simulink model "Scara"  (R2016b)
settings: Solver=VariableStepAuto  StartTime=0.0  StopTime=15.0  RelTol=1e-3
settings Model: Creator=Roozbeh  LastModifiedBy=Roozbeh

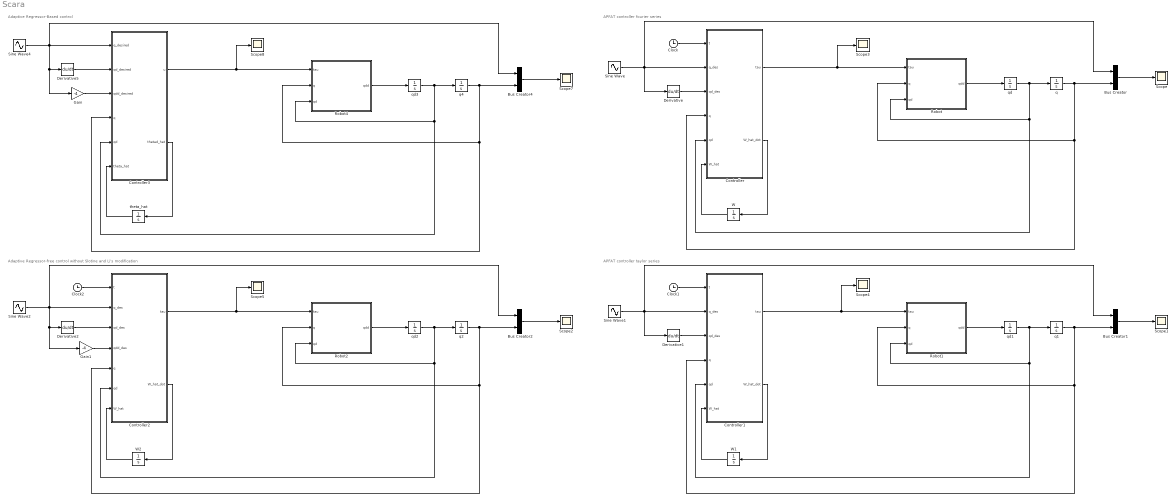
== system Scara ==
  note: Adaptive Regressor-free control without Slotine and Li's modification
  note: APFAT controller taylor series
  note: APFAT controller fourier series
  note: Adaptive Regressor-Based control
  Bus Creator{,1..2,4} (4 alike) : BusCreator  Inputs=2
  Clock : Clock
  Clock1 : Clock
  Clock2 : Clock
  Controller : MATLAB Function  TreatAsAtomicUnit=on
  Controller1 : MATLAB Function  TreatAsAtomicUnit=on
  Controller2 : MATLAB Function  TreatAsAtomicUnit=on
  Controller3 : MATLAB Function  TreatAsAtomicUnit=on
  Derivative{,1..2,5} (4 alike) : Derivative
  Gain : Gain  Gain=-4
  Gain1 : Gain  Gain=-4
  Robot : MATLAB Function  TreatAsAtomicUnit=on
  Robot1 : MATLAB Function  TreatAsAtomicUnit=on
  Robot2 : MATLAB Function  TreatAsAtomicUnit=on
  Robot4 : MATLAB Function  TreatAsAtomicUnit=on
  Scope{,1..5,7..8} (8 alike) : Scope
  Sine Wave{,1..2,4} (4 alike) : Sin  Amplitude=[1; 0.25; 0.5]  Bias=[0; 0 ; -pi/2]  Frequency=2  SampleTime=0
  W : Integrator  InitialCondition=zeros(3*9,3)
  W1 : Integrator  InitialCondition=zeros(3*3,3)
  W2 : Integrator  InitialCondition=zeros(3*3,3)
  q{,1..2,4} (4 alike) : Integrator  InitialCondition=[1.2; -1.2; 0.5]
  qd{,1..3} (4 alike) : Integrator  InitialCondition=zeros(3,1)
  theta_hat : Integrator  InitialCondition=|
      | [5.6542
      |     1.1574
      |     2.3321
      |     6.5314
      |     0.6524]'
  wires:
  Controller/1(tau) -> Scope3/1, Robot/1(tau)
  Controller/2(W_hat_dot) -> W/1
  W/1 -> Controller/6(W_hat)
  Robot/1(qdd) -> qd/1
  qd/1 -> Controller/5(qd), Robot/3(qd), q/1
  q/1 -> Bus Creator/2, Controller/4(q), Robot/2(q)
  Sine Wave/1 -> Bus Creator/1, Derivative/1, Controller/2(q_des)
  Derivative/1 -> Controller/3(qd_des)
  Clock/1 -> Controller/1(t)
  Bus Creator/1 -> Scope/1
  Controller1/1(tau) -> Scope4/1, Robot1/1(tau)
  Controller1/2(W_hat_dot) -> W1/1
  W1/1 -> Controller1/6(W_hat)
  Robot1/1(qdd) -> qd1/1
  qd1/1 -> q1/1, Robot1/3(qd), Controller1/5(qd)
  q1/1 -> Robot1/2(q), Controller1/4(q), Bus Creator1/2
  Sine Wave1/1 -> Controller1/2(q_des), Derivative1/1, Bus Creator1/1
  Derivative1/1 -> Controller1/3(qd_des)
  Clock1/1 -> Controller1/1(t)
  Bus Creator1/1 -> Scope1/1
  Controller2/1(tau) -> Scope5/1, Robot2/1(tau)
  Controller2/2(W_hat_dot) -> W2/1
  W2/1 -> Controller2/7(W_hat)
  Robot2/1(qdd) -> qd2/1
  qd2/1 -> Controller2/6(qd), Robot2/3(qd), q2/1
  q2/1 -> Bus Creator2/2, Controller2/5(q), Robot2/2(q)
  Sine Wave2/1 -> Bus Creator2/1, Gain1/1, Derivative2/1, Controller2/2(q_des)
  Derivative2/1 -> Controller2/3(qd_des)
  Clock2/1 -> Controller2/1(t)
  Bus Creator2/1 -> Scope2/1
  Controller3/1(u) -> Scope8/1, Robot4/1(tau)
  Controller3/2(thetad_hat) -> theta_hat/1
  theta_hat/1 -> Controller3/6(theta_hat)
  Robot4/1(qdd) -> qd3/1
  qd3/1 -> Controller3/5(qd), Robot4/3(qd), q4/1
  q4/1 -> Bus Creator4/2, Controller3/4(q), Robot4/2(q)
  Sine Wave4/1 -> Gain/1, Derivative5/1, Bus Creator4/1, Controller3/1(q_desired)
  Derivative5/1 -> Controller3/2(qd_desired)
  Bus Creator4/1 -> Scope7/1
  Gain/1 -> Controller3/3(qdd_desired)
  Gain1/1 -> Controller2/4(qdd_des)

== matlab function Scara/Controller1 ==
  data: t input; q_des input; qd_des input; q input; qd input; W_hat input; tau output; W_hat_dot output
function [tau, W_hat_dot] = fcn(t, q_des, qd_des, q, qd, W_hat)

gamma = diag([6 35 6]);
r = (qd - qd_des) + gamma * (q - q_des);

zz = [1; t; t^2];

Z = [zz' zz' zz']';

K = diag([300 3000 300]);

tau = transpose(W_hat)*Z - K*r;

% update
Q = 300*eye(3*3); % 3Bx3B
sigma = 0.009;

W_hat_dot = -pinv(Q)*(Z*transpose(r) + sigma*W_hat); %3Bx3

== matlab function Scara/Robot1 ==
  data: tau input; q input; qd input; qdd output
function qdd = fcn(tau, q, qd)

a1 = 0.6;
a2 = 0.4;

Lc1 = 0.3;
Lc2 = 0.2;

g = 9.81;
m1 = 12;
m2 = 6;
m3 = 6;
I1 = 0.36;
I2 = 0.36;
I3 = 0.36;

q1 = q(1);
q2 = q(2);
q3 = q(3);
qd1 = qd(1);
qd2 = qd(2);
qd3 = qd(3);

d11 = m1*Lc1^2 + m2*(a1^2 + Lc2^2 + 2*a1*Lc2*cos(q2)) + m3*(a1^2 + a2^2 + 2*a1*a2*cos(q2)) + I1 + I2 + I3;
d12 = m2*(Lc2^2 + a1*Lc2*cos(q2)) + m3*(a2^2 + a1*a2*cos(q2)) + I2 + I3;
d22 = m2*Lc2^2 + m3*a2^2 + I2 + I3;
d13 = 0;
d23 = 0;
d33 = m3;

D = [d11 d12 d13; d12 d22 d23; d13 d23 d33];

h = -m2*a1*Lc2*sin(q2) - m3*a1*a2*sin(q2);
C = [h*qd2 h*qd1+h*qd2 0; -h*qd1 0 0; 0 0 0];

G_mat = [0; 0; m3*g];

qdd = pinv(D)*(tau - C*qd - G_mat);

== matlab function Scara/Controller2 ==
  data: t input; q_des input; qd_des input; qdd_des input; q input; qd input; W_hat input; tau output; W_hat_dot output
function [tau, W_hat_dot] = fcn(t, q_des, qd_des, qdd_des, q, qd, W_hat)

e = q - q_des;
ed = qd - qd_des;

fn = 3;

zz = [1; cos(fn*t)*sin(fn*t); cos(2*fn*t)*sin(2*fn*t)];

Z = [zz; zz; zz]; % nB

Kd = diag([300 3000 300]);
Kp = diag([300 3000 300]);

tau = transpose(W_hat)*Z + qdd_des - Kp*e - Kd*ed;

% update
%Q = eye(2*3); % 2n x 2n
%A = [zeros(3) eye(3); -Kp, -Kd];
B = [zeros(3); eye(3)];
%P = lyap(A,Q)
P = [0.5017         0         0   -0.5000         0         0; ...
         0    0.5002         0         0   -0.5000         0; ...
         0         0    0.5017         0         0   -0.5000; ...
   -0.5000         0         0    0.5017         0         0; ...
         0   -0.5000         0         0    0.5002         0; ...
         0         0   -0.5000         0         0    0.5017];

gamma = 300*eye(3*3); % nB x nB
sigma = 0.009;
x = [e; ed];

W_hat_dot = -pinv(gamma)*(Z*transpose(x)*P*B + sigma*W_hat);

== matlab function Scara/Robot2 ==
  data: tau input; q input; qd input; qdd output
function qdd = fcn(tau, q, qd)

a1 = 0.6;
a2 = 0.4;

Lc1 = 0.3;
Lc2 = 0.2;

g = 9.81;
m1 = 12;
m2 = 6;
m3 = 6;
I1 = 0.36;
I2 = 0.36;
I3 = 0.36;

q1 = q(1);
q2 = q(2);
q3 = q(3);
qd1 = qd(1);
qd2 = qd(2);
qd3 = qd(3);

d11 = m1*Lc1^2 + m2*(a1^2 + Lc2^2 + 2*a1*Lc2*cos(q2)) + m3*(a1^2 + a2^2 + 2*a1*a2*cos(q2)) + I1 + I2 + I3;
d12 = m2*(Lc2^2 + a1*Lc2*cos(q2)) + m3*(a2^2 + a1*a2*cos(q2)) + I2 + I3;
d22 = m2*Lc2^2 + m3*a2^2 + I2 + I3;
d13 = 0;
d23 = 0;
d33 = m3;

D = [d11 d12 d13; d12 d22 d23; d13 d23 d33];

h = -m2*a1*Lc2*sin(q2) - m3*a1*a2*sin(q2);
C = [h*qd2 h*qd1+h*qd2 0; -h*qd1 0 0; 0 0 0];

G_mat = [0; 0; m3*g];

qdd = pinv(D)*(tau - C*qd - G_mat);

== matlab function Scara/Robot ==
  data: tau input; q input; qd input; qdd output
function qdd = fcn(tau, q, qd)

a1 = 0.6;
a2 = 0.4;

Lc1 = 0.3;
Lc2 = 0.2;

g = 9.81;
m1 = 12;
m2 = 6;
m3 = 6;
I1 = 0.36;
I2 = 0.36;
I3 = 0.36;

q1 = q(1);
q2 = q(2);
q3 = q(3);
qd1 = qd(1);
qd2 = qd(2);
qd3 = qd(3);

d11 = m1*Lc1^2 + m2*(a1^2 + Lc2^2 + 2*a1*Lc2*cos(q2)) + m3*(a1^2 + a2^2 + 2*a1*a2*cos(q2)) + I1 + I2 + I3;
d12 = m2*(Lc2^2 + a1*Lc2*cos(q2)) + m3*(a2^2 + a1*a2*cos(q2)) + I2 + I3;
d22 = m2*Lc2^2 + m3*a2^2 + I2 + I3;
d13 = 0;
d23 = 0;
d33 = m3;

D = [d11 d12 d13; d12 d22 d23; d13 d23 d33];

h = -m2*a1*Lc2*sin(q2) - m3*a1*a2*sin(q2);
C = [h*qd2 h*qd1+h*qd2 0; -h*qd1 0 0; 0 0 0];

G_mat = [0; 0; m3*g];

qdd = pinv(D)*(tau - C*qd - G_mat);

== matlab function Scara/Controller ==
  data: t input; q_des input; qd_des input; q input; qd input; W_hat input; tau output; W_hat_dot output
function [tau, W_hat_dot] = fcn(t, q_des, qd_des, q, qd, W_hat)

gamma = diag([6 35 6]);
r = (qd - qd_des) + gamma * (q - q_des);

fn = 10;
zz = [1; cos(fn*t)*sin(fn*t); cos(2*fn*t)*sin(2*fn*t); cos(3*fn*t)*sin(3*fn*t); cos(4*fn*t)*sin(4*fn*t);...
    cos(5*fn*t)*sin(5*fn*t); cos(6*fn*t)*sin(6*fn*t); cos(7*fn*t)*sin(7*fn*t); cos(8*fn*t)*sin(8*fn*t)];

Z = [zz' zz' zz']';

K = diag([300 3000 300]);

tau = transpose(W_hat)*Z - K*r;

% update
Q = 300*eye(3*9); % 3Bx3B
sigma = 0.009;

W_hat_dot = -pinv(Q)*(Z*transpose(r) + sigma*W_hat); %3Bx3

== matlab function Scara/Controller3 ==
  data: q_desired input; qd_desired input; qdd_desired input; q input; qd input; theta_hat input; u output; thetad_hat output
function [u, thetad_hat] = fcn(q_desired, qd_desired, qdd_desired, q, qd,theta_hat)

g = 9.81;
q1 = q(1);
q2 = q(2);
q3 = q(3);

qd1 = qd(1);
qd2 = qd(2);
qd3 = qd(3);

e_q = q - q_desired;
e_qd = qd - qd_desired;

gamma = eye(3);
v = qd_desired - gamma*e_q;
vd = qdd_desired - gamma*e_qd;
r = qd - v;

wn = 10;
Kd = eye(3)*wn^2;
Kp = eye(3)*2*wn;
qdd1 = vd(1);
qdd2 = vd(2);
qdd3 = vd(3);

Y = [qdd1 qdd1 + qdd2 2*qdd1*cos(q2) + qdd2*cos(q2) - v(1)*qd2*sin(q2) - qd1*v(2)*sin(q2) - 2*qd2*v(2)*sin(q2) 0 qdd1 + qdd2; ...
    0 qdd1 + qdd2 qdd1*cos(q2) + qd1*v(1)*sin(q2) 0 qdd1 + qdd2; 0 0 0 qdd3 + g 0];

K = 5*eye(3);
u = Y*theta_hat - K*r;

%update
L = eye(5)*2;
thetad_hat = -pinv(L)*transpose(Y)*r;

== matlab function Scara/Robot4 ==
  data: tau input; q input; qd input; qdd output
function qdd = fcn(tau, q, qd)

a1 = 0.6;
a2 = 0.4;

Lc1 = 0.3;
Lc2 = 0.2;

g = 9.81;
m1 = 12;
m2 = 6;
m3 = 6;
I1 = 0.36;
I2 = 0.36;
I3 = 0.36;

q1 = q(1);
q2 = q(2);
q3 = q(3);
qd1 = qd(1);
qd2 = qd(2);
qd3 = qd(3);

d11 = m1*Lc1^2 + m2*(a1^2 + Lc2^2 + 2*a1*Lc2*cos(q2)) + m3*(a1^2 + a2^2 + 2*a1*a2*cos(q2)) + I1 + I2 + I3;
d12 = m2*(Lc2^2 + a1*Lc2*cos(q2)) + m3*(a2^2 + a1*a2*cos(q2)) + I2 + I3;
d22 = m2*Lc2^2 + m3*a2^2 + I2 + I3;
d13 = 0;
d23 = 0;
d33 = m3;

D = [d11 d12 d13; d12 d22 d23; d13 d23 d33];

h = -m2*a1*Lc2*sin(q2) - m3*a1*a2*sin(q2);
C = [h*qd2 h*qd1+h*qd2 0; -h*qd1 0 0; 0 0 0];

G_mat = [0; 0; m3*g];

qdd = pinv(D)*(tau - C*qd - G_mat);
